simulink model "Simulation"  (Simulink 7.7)
settings: Solver=ode1  StartTime=0.0  StopTime=50  FixedStep=0.002  RelTol=1e-3
values from neighbouring files (symbols this model uses):
  A = zeros(4,4)    [Setup_sim.m]
  B = zeros(4,1)    [Setup_sim.m]
  C = zeros(2,4)    [Setup_sim.m]
  D = zeros(2,1)    [Setup_sim.m]
  K_AMP = 1    [Setup_sim.m]
  K_CT = lqr(Ai,Bi,Qx,Qu)    [Setup_sim.m]
  sysc = ss(A,B,C,D)    [Setup_sim.m]
  VMAX_DAC = 10    [Setup_sim.m]
undefined symbols (not defined in the file or in its folder): DiscIntNeverNeededParam, L_CT, VMAX_AMP
libraries: simulink_extras x7
settings Model: Creator=MLevis  LastModifiedBy=Ramin_hp  ExtModeTrigDuration=10000
settings SolverCC: PositivePriorityOrder=on
settings OptimizationCC: BooleanDataType=off  OptimizeBlockIOStorage=off  BufferReuse=off  ExpressionFolding=off  LocalBlockOutputs=off  InitFltsAndDblsToZero=on
settings DebuggingCC: SaveWithParameterizedLinksMsg=none  SignalResolutionControl=TryResolveAllWithWarning  SolverPrmCheckMsg=none  MultiTaskDSMMsg=warning  MultiTaskCondExecSysMsg=none
settings HardwareCC: TargetHWDeviceType=32-bit Generic
settings RTWCC: SystemTargetFile=quarc_windows.tlc  TemplateMakefile=quarc_default_tmf  Description=Quarc Win32 Target
settings CodeAppCC: CustomSymbolStrType=$N$R$M_T
settings STFCustomTargetCC: TargetFcnLib=ansi_tfl_tmw.mat  TargetPreCompLibLocation=C:\PROGRA~3\QUARC\lib\2015a\windows\release  TargetFunctionLibrary=C89/C90 (ANSI)  GeneratePreprocessorConditionals=Disable all  SystemTargetFile=quarc_windows.tlc
settings GRTTargetCC: TargetFcnLib=ansi_tfl_tmw.mat  TargetPreCompLibLocation=C:\PROGRA~3\QUARC\lib\2015a\windows\release  TargetFunctionLibrary=C89/C90 (ANSI)  ParMdlRefBuildCompliant=off  CompOptLevelCompliant=off  MatFileLogging=off  ExtMode=on  ExtModeMexFile=quarc_comm

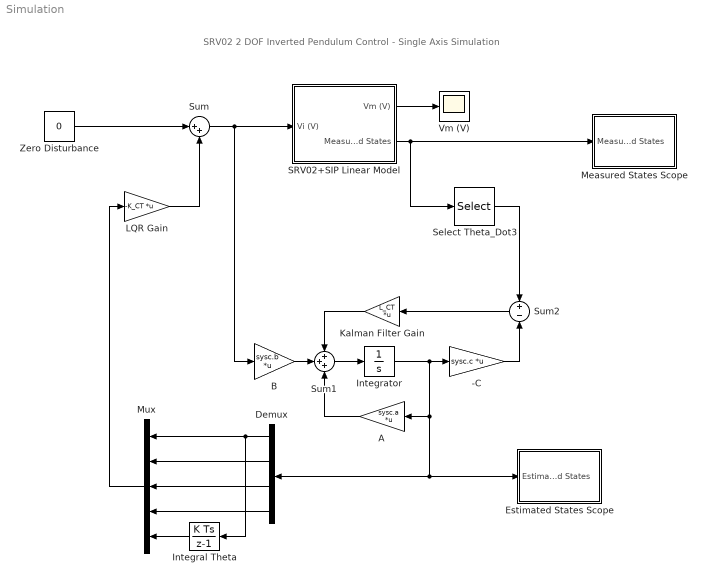
== system Simulation ==
  note: SRV02 2 DOF Inverted Pendulum Control - Single Axis Simulation
  -C : Gain  Gain=sysc.c  Multiplication=Matrix(K*u)
  A : Gain  Gain=sysc.a  Multiplication=Matrix(K*u)
  B : Gain  Gain=sysc.b  Multiplication=Matrix(K*u)
  Demux : Demux
  Estimated States Scope : Subsystem
  Integral Theta : DiscreteIntegrator  SampleTime=0.002  ICPrevOutput=DiscIntNeverNeededParam  ICPrevScaledInput=DiscIntNeverNeededParam
  Integrator : Integrator
  Kalman Filter Gain : Gain  Gain=L_CT  Multiplication=Matrix(K*u)
  LQR Gain : Gain  Gain=-K_CT  Multiplication=Matrix(K*u)  SaturateOnIntegerOverflow=on  OutDataTypeStr=Inherit: Same as input  ParamDataTypeStr=Inherit: Same as input
  Measured States Scope : Subsystem
  Mux : Mux  Inputs=5
  SRV02+SIP Linear Model : Subsystem
  Select Theta_Dot3 : Selector  InputPortWidth=3  IndexOptions=Index vector (dialog)  Indices=[1 2]  OutputSizes=1
  Sum : Sum  Inputs=|++
  Sum1 : Sum  Inputs=+++
  Sum2 : Sum  Inputs=+|-
  Vm (V) : Scope
      settings: TimeRange=5  TickLabels=on  MaxDataPoints=5000  SaveToWorkspace=off  SaveName=data_vm  YMin=-1.17798  YMax=1.242  SampleTime=-1  DataFormat=Array
  Zero Disturbance : Constant  Value=0
  wires:
  LQR Gain/1 -> Sum/2
  B/1 -> Sum1/2
  Sum1/1 -> Integrator/1
  Integrator/1 -> Demux/1, Estimated States Scope/1(Estimated States), A/1, -C/1
  -C/1 -> Sum2/2
  Sum2/1 -> Kalman Filter Gain/1
  Kalman Filter Gain/1 -> Sum1/1
  A/1 -> Sum1/3
  Sum/1 -> SRV02+SIP Linear Model/1(Vi (V)), B/1
  SRV02+SIP Linear Model/2(Measured States) -> Measured States Scope/1(Measured States), Select Theta_Dot3/1
  SRV02+SIP Linear Model/1(Vm (V)) -> Vm (V)/1
  Zero Disturbance/1 -> Sum/1
  Select Theta_Dot3/1 -> Sum2/1
  Demux/1 -> Integral Theta/1, Mux/1
  Demux/2 -> Mux/2
  Demux/3 -> Mux/3
  Demux/4 -> Mux/4
  Mux/1 -> LQR Gain/1
  Integral Theta/1 -> Mux/5

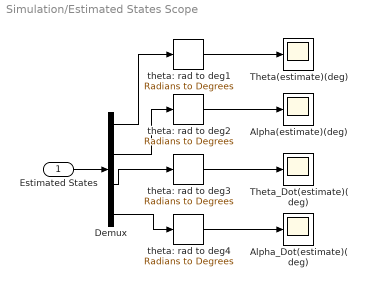
== system Simulation/Estimated States Scope ==
  Estimated States : Inport
  Alpha(estimate)(deg) : Scope
      settings: TimeRange=5  MaxDataPoints=5000  SaveToWorkspace=off  SaveName=data_alpha3  YMin=-9.5e-07  YMax=-4.5e-07  SampleTime=-1  DataFormat=Array
  Alpha_Dot(estimate)(deg) : Scope
      settings: TimeRange=5  MaxDataPoints=5000  SaveToWorkspace=off  SaveName=data_alpha  YMin=-962986.15119  YMax=8666875.3607  SampleTime=-1  DataFormat=Array
  Demux : Demux
  Theta(estimate)(deg) : Scope
      settings: TimeRange=300  MaxDataPoints=5000  SaveToWorkspace=off  SaveName=data_theta2  YMin=-17074.06908  YMax=153616.62176  SampleTime=-1  DataFormat=Array
  Theta_Dot(estimate)(deg) : Scope
      settings: TimeRange=5  MaxDataPoints=5000  SaveToWorkspace=off  SaveName=data_alpha4  YMin=-119395.41536  YMax=1074558.73827  SampleTime=-1  DataFormat=Array
  theta: rad to deg{1..4} (4 alike) : simulink_extras/Transformations/Radians to Degrees
  wires:
  Demux/1 -> theta: rad to deg1/1
  theta: rad to deg1/1 -> Theta(estimate)(deg)/1
  theta: rad to deg2/1 -> Alpha(estimate)(deg)/1
  Demux/2 -> theta: rad to deg2/1
  theta: rad to deg3/1 -> Theta_Dot(estimate)(deg)/1
  Demux/3 -> theta: rad to deg3/1
  theta: rad to deg4/1 -> Alpha_Dot(estimate)(deg)/1
  Demux/4 -> theta: rad to deg4/1
  Estimated States/1 -> Demux/1

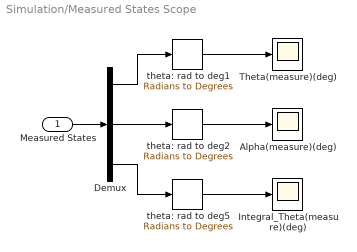
== system Simulation/Measured States Scope ==
  Measured States : Inport
  Alpha(measure)(deg) : Scope
      settings: TimeRange=5  MaxDataPoints=5000  SaveToWorkspace=off  SaveName=data_alpha3  YMin=0.000000211  YMax=0.000000279  SampleTime=-1  DataFormat=Array
  Demux : Demux  Outputs=3
  Integral_Theta(measure)(deg) : Scope
      settings: TimeRange=5  MaxDataPoints=5000  SaveToWorkspace=off  SaveName=data_alpha2  YMin=0.18213  YMax=0.24097  SampleTime=-1  DataFormat=Array
  Theta(measure)(deg) : Scope
      settings: TimeRange=50  MaxDataPoints=5000  SaveToWorkspace=off  SaveName=data_theta2  YMin=-20.93974  YMax=15.53818  SampleTime=-1  DataFormat=Array
  theta: rad to deg1 : simulink_extras/Transformations/Radians to Degrees
  theta: rad to deg2 : simulink_extras/Transformations/Radians to Degrees
  theta: rad to deg5 : simulink_extras/Transformations/Radians to Degrees
  wires:
  Measured States/1 -> Demux/1
  theta: rad to deg5/1 -> Integral_Theta(measure)(deg)/1
  theta: rad to deg2/1 -> Alpha(measure)(deg)/1
  theta: rad to deg1/1 -> Theta(measure)(deg)/1
  Demux/1 -> theta: rad to deg1/1
  Demux/2 -> theta: rad to deg2/1
  Demux/3 -> theta: rad to deg5/1

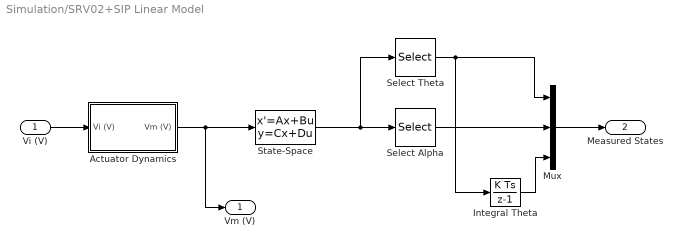
== system Simulation/SRV02+SIP Linear Model ==
  Vi (V) : Inport
  Actuator Dynamics : Subsystem
  Integral Theta : DiscreteIntegrator  SampleTime=0.002  ICPrevOutput=DiscIntNeverNeededParam  ICPrevScaledInput=DiscIntNeverNeededParam
  Mux : Mux  Inputs=3
  Select Alpha : Selector  InputPortWidth=2  IndexOptions=Index vector (dialog)  Indices=2  OutputSizes=1
  Select Theta : Selector  InputPortWidth=2  IndexOptions=Index vector (dialog)  Indices=1  OutputSizes=1
  State-Space : StateSpace  A=A  B=B  C=C  D=D  X0=pi/180*[-5, 2, 4, 0.3]
  Vm (V) : Outport
  Measured States : Outport  Port=2
  wires:
  Vi (V)/1 -> Actuator Dynamics/1(Vi (V))
  Actuator Dynamics/1(Vm (V)) -> State-Space/1, Vm (V)/1
  Mux/1 -> Measured States/1
  Integral Theta/1 -> Mux/3
  Select Alpha/1 -> Mux/2
  Select Theta/1 -> Mux/1, Integral Theta/1
  State-Space/1 -> Select Alpha/1, Select Theta/1

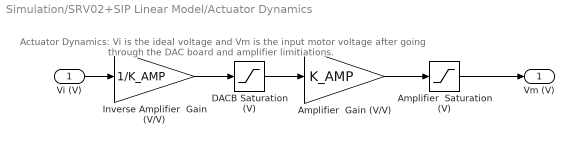
== system Simulation/SRV02+SIP Linear Model/Actuator Dynamics ==
  note: Actuator Dynamics: Vi is the ideal voltage and Vm is the
      | input motor voltage after going through the DAC board and amplifier limitiations.
  Vi (V) : Inport
  Amplifier  Gain (V/V) : Gain  Gain=K_AMP
  Amplifier  Saturation (V) : Saturate  UpperLimit=VMAX_AMP  LowerLimit=-VMAX_AMP
  DACB Saturation (V) : Saturate  UpperLimit=VMAX_DAC  LowerLimit=-VMAX_DAC
  Inverse Amplifier  Gain (V/V) : Gain  Gain=1/K_AMP
  Vm (V) : Outport
  wires:
  Inverse Amplifier  Gain (V/V)/1 -> DACB Saturation (V)/1
  DACB Saturation (V)/1 -> Amplifier  Gain (V/V)/1
  Amplifier  Gain (V/V)/1 -> Amplifier  Saturation (V)/1
  Vi (V)/1 -> Inverse Amplifier  Gain (V/V)/1
  Amplifier  Saturation (V)/1 -> Vm (V)/1
